simulink model "lqrControl"  (R2017b)
settings: Solver=FixedStepAuto  StartTime=0.0  StopTime=10.0  FixedStep=1e-2  RelTol=1e-3
values from neighbouring files (symbols this model uses):
  Klqr = designLQR(A2, B2, Q, R)    [calcSystem.m]
settings Model: Creator=Haotian  LastModifiedBy=Haotian

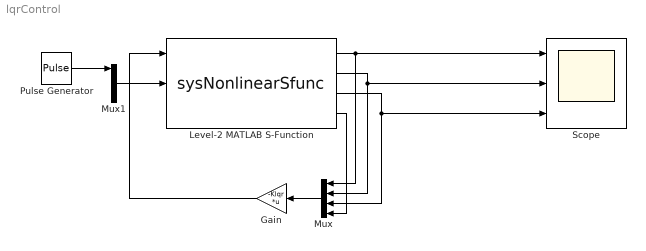
== system lqrControl ==
  Gain : Gain  Gain=-Klqr  Multiplication=Matrix(K*u)
  Level-2 MATLAB S-Function : M-S-Function  FunctionName=sysNonlinearSfunc  Parameters=Mc, Mg, b, l, I, init_phi, useAcc  mask(S-function: sysNonlinearSfunc){Mc=1.096, Mg=0.109, b=0.1, l=0.25, I=0.0034, init_phi=0.01, useAcc=on}
      mask prompts: Mc "小车质量"; Mg "摆杆质量"; b "小车摩擦系数"; l "摆杆转动轴心到杆质心的长度"; I "摆杆惯量"; init_phi "初始垂直夹角"; useAcc "使用加速度作为输入"
      mask help: 一阶倒立摆非线性模型。
      mask Display:
      | fprintf('一阶倒立摆\n\nM=%.3f m=%.3f\nb=%.3f l=%.3f\nI=%.3f phi0=%.2f\n\nX=[x dx phi dphi]', Mc, Mg, b, l, I, init_phi);
      | if(useAcc)
      |     port_label('input', 1, 'a');
      | else
      |     port_label('input', 1, 'F');
      | end
      | port_label('input', 2, 'setX');
      | port_label('input', 3, 'devX');
      | 
      | port_label('output', 1, 'x');
      | port_label('output', 2, 'v');
      | port_label('output', 3, '\phi','texmode','on');
      | port_label('output', 4, 'd\phi','texmode','on');
  Mux : Mux
  Mux1 : Mux
  Pulse Generator : DiscretePulseGenerator  PulseType=Time based  Period=10  PhaseDelay=1
  Scope : Scope  NumInputPorts=3
  wires:
  Level-2 MATLAB S-Function/3 -> Mux/3, Scope/3
  Level-2 MATLAB S-Function/1 -> Mux/1, Scope/1
  Level-2 MATLAB S-Function/2 -> Mux/2, Scope/2
  Level-2 MATLAB S-Function/4 -> Mux/4
  Mux/1 -> Gain/1
  Gain/1 -> Level-2 MATLAB S-Function/1
  Mux1/1 -> Level-2 MATLAB S-Function/2
  Pulse Generator/1 -> Mux1/1
